simulink model "BSCForFiveAxisExperiment01"  (Simulink 8.4)
settings: Solver=ode1  StartTime=0.0  StopTime=5.122  FixedStep=0.001  RelTol=1e-3
InitFcn:
  | MainContourControlExp
values from neighbouring files (symbols this model uses):
  Acommands = DriveCommands(:,4)-HomePosDrive(4)    [MainContourControlExp.m]
  c1_i = 0.2    [MainContourControlExp.m]
  c1_j = c1_i    (= 0.2)    [MainContourControlExp.m]
  c1_k = c1_i    (= 0.2)    [MainContourControlExp.m]
  c1_x = 2    [MainContourControlExp.m]
  c1_y = c1_x    (= 2)    [MainContourControlExp.m]
  c1_z = c1_x    (= 2)    [MainContourControlExp.m]
  Ccommands = DriveCommands(:,5)-HomePosDrive(5)    [MainContourControlExp.m]
  k_i = 0.2    [MainContourControlExp.m]
  k_j = k_i    (= 0.2)    [MainContourControlExp.m]
  k_k = k_i    (= 0.2)    [MainContourControlExp.m]
  k_x = 1    [MainContourControlExp.m]
  k_y = k_x    (= 1)    [MainContourControlExp.m]
  k_z = k_x    (= 1)    [MainContourControlExp.m]
  PlantADen = [1 PlantAPara.a1 PlantAPara.a0]    [MainContourControlExp.m]
  PlantANum = [PlantAPara.b1 PlantAPara.b0]    [MainContourControlExp.m]
  PlantCDen = [1 PlantCPara.a1 PlantCPara.a0]    [MainContourControlExp.m]
  PlantCNum = [PlantCPara.b1 PlantCPara.b0]    [MainContourControlExp.m]
  PlantXDen = [1 PlantXPara.a1 PlantXPara.a0]    [MainContourControlExp.m]
  PlantXNum = [PlantXPara.b1 PlantXPara.b0]    [MainContourControlExp.m]
  PlantYDen = [1 PlantYPara.a1 PlantYPara.a0]    [MainContourControlExp.m]
  PlantYNum = [PlantYPara.b1 PlantYPara.b0]    [MainContourControlExp.m]
  PlantZDen = [1 PlantZPara.a1 PlantZPara.a0]    [MainContourControlExp.m]
  PlantZNum = [PlantZPara.b1 PlantZPara.b0]    [MainContourControlExp.m]
  R1 = 0.8    [MainContourControlExp.m]
  R2 = R1    (= 0.8)    [MainContourControlExp.m]
  R3 = R1    (= 0.8)    [MainContourControlExp.m]
  R4 = 0.8    [MainContourControlExp.m]
  R5 = R4    (= 0.8)    [MainContourControlExp.m]
  R6 = R4    (= 0.8)    [MainContourControlExp.m]
  Ts = 0.001    [MainContourControlExp.m]
  VlimitA = 5    [MainContourControlExp.m]
  VlimitC = 5    [MainContourControlExp.m]
  VlimitX = 6    [MainContourControlExp.m]
  VlimitY = 6    [MainContourControlExp.m]
  VlimitZ = 6    [MainContourControlExp.m]
  Xcommands = DriveCommands(:,1)-HomePosDrive(1)    [MainContourControlExp.m]
  Ycommands = DriveCommands(:,2)-HomePosDrive(2)    [MainContourControlExp.m]
  Zcommands = DriveCommands(:,3)-HomePosDrive(3)    [MainContourControlExp.m]
libraries: simulink x8
settings Model: Creator=Administrator  LastModifiedBy=Administrator
settings DataIOCC: SignalLoggingSaveFormat=Dataset
settings OptimizationCC: ExpressionDepthLimit=128
settings DebuggingCC: UnderspecifiedInitializationDetection=Simplified  MergeDetectMultiDrivingBlocksExec=error  FcnCallInpInsideContextMsg=EnableAllAsError  StateNameClashWarn=none
settings GRTTargetCC: CombineOutputUpdateFcns=on  GRTInterface=off

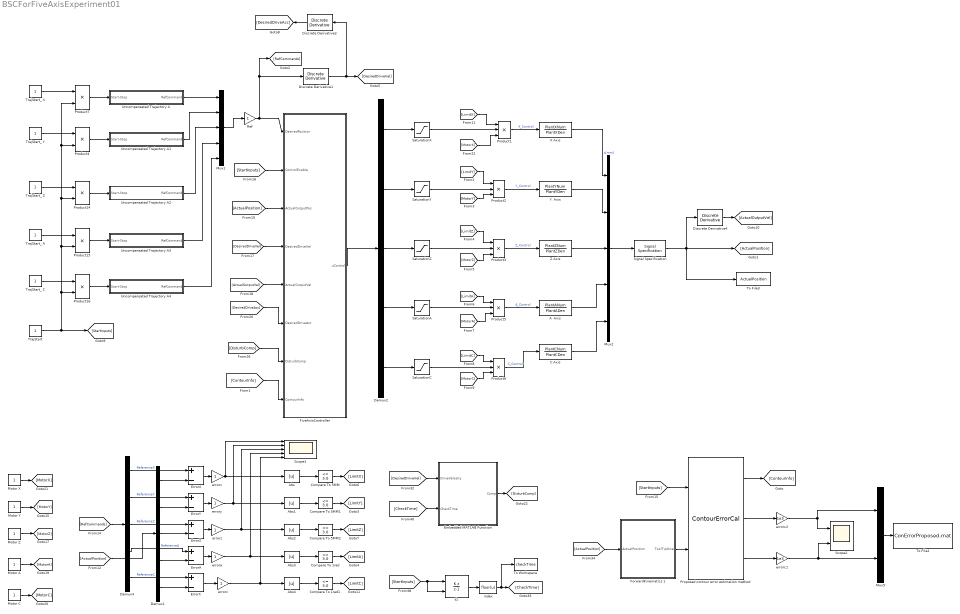
== system BSCForFiveAxisExperiment01 ==
  A  Axis : DiscreteTransferFcn  Numerator=PlantANum  Denominator=PlantADen  SampleTime=Ts
  Abs{,1..4} (5 alike) : Abs
  C Axis : DiscreteTransferFcn  Numerator=PlantCNum  Denominator=PlantCDen  SampleTime=Ts
  Compare To 1rad : simulink/Logic and Bit Operations/Compare To Constant  relop=<=  const=3.0  OutDataTypeStr=boolean
  Compare To 1rad1 : simulink/Logic and Bit Operations/Compare To Constant  relop=<=  const=3.0  OutDataTypeStr=boolean
  Compare To 5MM : simulink/Logic and Bit Operations/Compare To Constant  relop=<=  const=3.0  OutDataTypeStr=boolean
  Compare To 5MM1 : simulink/Logic and Bit Operations/Compare To Constant  relop=<=  const=3.0  OutDataTypeStr=boolean
  Compare To 5MM2 : simulink/Logic and Bit Operations/Compare To Constant  relop=<=  const=3.0  OutDataTypeStr=boolean
  Demux1 : Demux  Outputs=5
  Demux2 : Demux  Outputs=5
  Demux4 : Demux  Outputs=5
  Discrete Derivative1 : simulink/Discrete/Discrete Derivative  gainval=1.0  ICPrevScaledInput=0.0  InputProcessing=Inherited  OutMin=[]  OutMax=[]  OutDataType=fixdt(1, 16)  OutScaling=2^-10  DoSatur=off
  Discrete Derivative2 : simulink/Discrete/Discrete Derivative  gainval=1.0  ICPrevScaledInput=0.0  InputProcessing=Inherited  OutMin=[]  OutMax=[]  OutDataType=fixdt(1, 16)  OutScaling=2^-10  DoSatur=off
  Discrete Derivative4 : simulink/Discrete/Discrete Derivative  gainval=1.0  ICPrevScaledInput=0.0  InputProcessing=Inherited  OutMin=[]  OutMax=[]  OutDataType=fixdt(1, 16)  OutScaling=2^-10  DoSatur=off
  Embedded MATLAB Function : MATLAB Function  TreatAsAtomicUnit=on
  ErrorA : Sum  Inputs=+-
  ErrorC : Sum  Inputs=+-
  ErrorX : Sum  Inputs=+-
  ErrorY : Sum  Inputs=+-
  ErrorZ : Sum  Inputs=+-
  FiveAxisController : MATLAB Function  TreatAsAtomicUnit=on
  ForwardKinematics 1 : MATLAB Function  TreatAsAtomicUnit=on
  Motor A : Constant
  Motor C : Constant
  Motor X : Constant
  Motor Y : Constant
  Motor Z : Constant
  Mux1 : Mux  Inputs=5
  Mux2 : Mux  Inputs=5
  Mux5 : Mux  Inputs=2
  Product{1..3,5..6} (5 alike) : Product  Inputs=3  RndMeth=Zero
  Product{4,7,14..16} (5 alike) : Product  SampleTime=Ts  RndMeth=Zero
  Proposed contour error estimation method : S-Function  FunctionName=ContourErrorCal  Parameters=X Y Z I J K U  EnableBusSupport=off
  "Ref " : Gain  SampleTime=0.001
  SaturationA : Saturate  UpperLimit=VlimitA  LowerLimit=-VlimitA
  SaturationC : Saturate  UpperLimit=VlimitC  LowerLimit=-VlimitC
  SaturationX : Saturate  UpperLimit=VlimitX  LowerLimit=-VlimitX
  SaturationY : Saturate  UpperLimit=VlimitY  LowerLimit=-VlimitY
  SaturationZ : Saturate  UpperLimit=VlimitZ  LowerLimit=-VlimitZ
  Scope1 : Scope  NumInputPorts=5
      settings: TimeRange=5.122  YMin=-0.1~-0.04~-0.04~-0.001~-0.0015  YMax=0.1~0.06~0.06~0.001~0.0015  SaveName=ScopeData2  MaxDataPoints=5122
  Scope2 : Scope  NumInputPorts=2
      settings: YMin=0~0  YMax=90~1.2  SaveName=ScopeData3
  Signal Specification : SignalSpecification  Dimensions=5
  To File2 : ToFile  Filename=ConErrorProposed.mat  MatrixName=Proposed
  To File3 : ToFile  Filename=ActualPosition  MatrixName=ActualPos
  To Workspace : ToWorkspace  VariableName=checkTime  SampleTime=-1
  TrajStart : Constant
  TrajStart_ A : Constant
  TrajStart_ C : Constant
  "TrajStart_ X " : Constant
  TrajStart_ Y : Constant
  TrajStart_ Z : Constant
  Uncompensated Trajectory A : Subsystem
  Uncompensated Trajectory A1 : Subsystem
  Uncompensated Trajectory A2 : Subsystem
  Uncompensated Trajectory A3 : Subsystem
  Uncompensated Trajectory A4 : Subsystem
  "X Axis " : DiscreteTransferFcn  Numerator=PlantXNum  Denominator=PlantXDen  SampleTime=Ts
  Y  Axis : DiscreteTransferFcn  Numerator=PlantYNum  Denominator=PlantYDen  SampleTime=Ts
  Z Axis : DiscreteTransferFcn  Numerator=PlantZNum  Denominator=PlantZDen  SampleTime=Ts
  errora : Gain  SampleTime=0.001
  errorc : Gain  SampleTime=0.001
  errorc1 : Gain  Gain=1e3  SampleTime=0.001
  errorc2 : Gain  Gain=1e3  SampleTime=0.001
  errorx : Gain  SampleTime=0.001
  errory : Gain  SampleTime=0.001
  errorz : Gain  SampleTime=0.001
  index : Fcn  Expr=floor(u)
  t1 : DiscreteIntegrator  IntegratorMethod=Accumulation: Backward Euler  ExternalReset=rising  SampleTime=Ts
  wires:
  TrajStart/1 -> [StartInputs], Product16/2, Product15/2, Product14/2, Product7/2, Product4/2
  SaturationX/1 -> Product1/2
  [LimitX] -> Product1/1
  [MotorX] -> Product1/3
  Product1/1 -> "X Axis "/1  "X_Control"
  Mux1/1 -> "Ref "/1
  SaturationY/1 -> Product2/2
  [LimitY] -> Product2/1
  [MotorY] -> Product2/3
  Product2/1 -> Y  Axis/1  "Y_Control"
  SaturationZ/1 -> Product3/2
  [LimitZ] -> Product3/1
  [MotorZ] -> Product3/3
  Product3/1 -> Z Axis/1  "Z_Control"
  SaturationA/1 -> Product5/2
  [LimitA] -> Product5/1
  [MotorA] -> Product5/3
  Product5/1 -> A  Axis/1  "A_Control"
  SaturationC/1 -> Product6/2
  [LimitC] -> Product6/1
  [MotorC] -> Product6/3
  Product6/1 -> C Axis/1  "C_Control"
  Compare To 5MM/1 -> [LimitX]
  Abs/1 -> Compare To 5MM/1
  Compare To 5MM1/1 -> [LimitY]
  Abs1/1 -> Compare To 5MM1/1
  ErrorY/1 -> errory/1
  Demux1/1 -> ErrorX/2
  Demux1/2 -> ErrorY/2
  Demux4/1 -> ErrorX/1  "ReferenceX"
  Demux4/2 -> ErrorY/1  "ReferenceY"
  [RefCommands] -> Demux4/1
  Compare To 5MM2/1 -> [LimitZ]
  Abs2/1 -> Compare To 5MM2/1
  ErrorZ/1 -> errorz/1
  Demux1/3 -> ErrorZ/2
  Demux4/3 -> ErrorZ/1  "ReferenceZ"
  Compare To 1rad/1 -> [LimitA]
  Abs3/1 -> Compare To 1rad/1
  Demux1/4 -> ErrorA/2
  Demux4/4 -> ErrorA/1  "ReferenceA"
  Compare To 1rad1/1 -> [LimitC]
  Abs4/1 -> Compare To 1rad1/1
  ErrorC/1 -> errorc/1
  Demux1/5 -> ErrorC/2
  Demux4/5 -> ErrorC/1  "ReferenceC"
  [ActualPosition] -> Demux1/1
  Discrete Derivative1/1 -> [DesiredDriveVel], Discrete Derivative2/1
  Discrete Derivative2/1 -> [DesiredDriveAcc]
  t1/1 -> index/1
  [StartInputs] -> t1/1, t1/2
  index/1 -> To Workspace/1, [CheckTime]
  Embedded MATLAB Function/1(Comp) -> [DisturbComp]
  [DesiredDriveVel] -> Embedded MATLAB Function/1(DriveVelosity)
  [CheckTime] -> Embedded MATLAB Function/2(CheckTime)
  ErrorA/1 -> errora/1
  ErrorX/1 -> errorx/1
  "TrajStart_ X "/1 -> Product7/1
  "Ref "/1 -> [RefCommands], Discrete Derivative1/1, FiveAxisController/1(DesiredPosition)
  errorx/1 -> Scope1/1, Abs/1
  errory/1 -> Scope1/2, Abs1/1
  errorz/1 -> Scope1/3, Abs2/1
  errora/1 -> Scope1/4, Abs3/1
  errorc/1 -> Scope1/5, Abs4/1
  Product7/1 -> Uncompensated Trajectory A/1(Start-Stop)
  Product4/1 -> Uncompensated Trajectory A1/1(Start-Stop)
  Product14/1 -> Uncompensated Trajectory A2/1(Start-Stop)
  Product15/1 -> Uncompensated Trajectory A3/1(Start-Stop)
  TrajStart_ Y/1 -> Product4/1
  TrajStart_ Z/1 -> Product14/1
  TrajStart_ A/1 -> Product15/1
  TrajStart_ C/1 -> Product16/1
  Product16/1 -> Uncompensated Trajectory A4/1(Start-Stop)
  Uncompensated Trajectory A3/1(RefCommand) -> Mux1/4
  Uncompensated Trajectory A/1(RefCommand) -> Mux1/1
  Uncompensated Trajectory A1/1(RefCommand) -> Mux1/2
  Uncompensated Trajectory A2/1(RefCommand) -> Mux1/3
  Uncompensated Trajectory A4/1(RefCommand) -> Mux1/5
  [StartInputs] -> FiveAxisController/2(ControlEnable)
  [ActualPosition] -> FiveAxisController/3(ActualOutputPos)
  [DesiredDriveVel] -> FiveAxisController/4(DesiredDriveVel)
  [DesiredDriveAcc] -> FiveAxisController/6(DesiredDriveAcc)
  [ActualOutputVel] -> FiveAxisController/5(ActualOutputVel)
  [DisturbComp] -> FiveAxisController/7(DisturbComp)
  [ContourInfo] -> FiveAxisController/8(ContourInfo)
  FiveAxisController/1(uControl) -> Demux2/1
  Demux2/5 -> SaturationC/1
  Demux2/4 -> SaturationA/1
  Demux2/3 -> SaturationZ/1
  Demux2/2 -> SaturationY/1
  Demux2/1 -> SaturationX/1
  Discrete Derivative4/1 -> [ActualOutputVel]
  Mux2/1 -> Signal Specification/1
  Signal Specification/1 -> Discrete Derivative4/1, To File3/1, [ActualPosition]
  "X Axis "/1 -> Mux2/1  "x[mm]"
  Y  Axis/1 -> Mux2/2
  Z Axis/1 -> Mux2/3
  A  Axis/1 -> Mux2/4
  C Axis/1 -> Mux2/5
  Motor Y/1 -> [MotorY]
  Motor X/1 -> [MotorX]
  Motor Z/1 -> [MotorZ]
  Motor A/1 -> [MotorA]
  Motor C/1 -> [MotorC]
  [StartInputs] -> Proposed contour error estimation method/1
  ForwardKinematics 1/1(ToolTipOrien) -> Proposed contour error estimation method/2
  Proposed contour error estimation method/1 -> [ContourInfo]
  [ActualPosition] -> ForwardKinematics 1/1(ActualPosition)
  Proposed contour error estimation method/2 -> errorc2/1
  Proposed contour error estimation method/3 -> errorc1/1
  Mux5/1 -> To File2/1
  errorc2/1 -> Mux5/1, Scope2/1
  errorc1/1 -> Mux5/2, Scope2/2

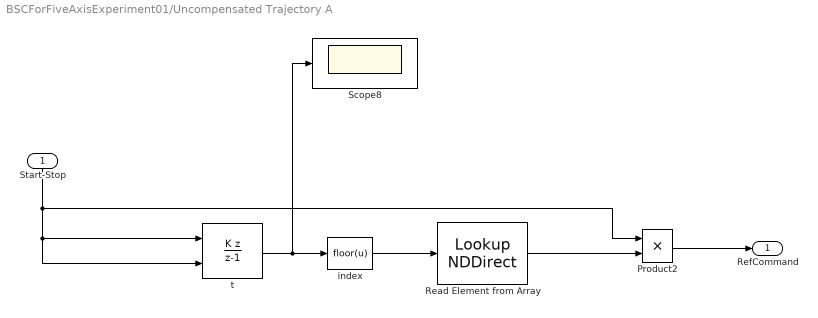
== system BSCForFiveAxisExperiment01/Uncompensated Trajectory A ==
  Start-Stop : Inport
  Product2 : Product  RndMeth=Zero
  Read Element from Array : LookupNDDirect  NumberOfTableDimensions=1  Table=Xcommands
  Scope8 : Scope
  index : Fcn  Expr=floor(u)
  t : DiscreteIntegrator  IntegratorMethod=Accumulation: Backward Euler  ExternalReset=rising  SampleTime=Ts
  RefCommand : Outport
  wires:
  Read Element from Array/1 -> Product2/2
  t/1 -> Scope8/1, index/1
  Product2/1 -> RefCommand/1
  Start-Stop/1 -> Product2/1, t/1, t/2
  index/1 -> Read Element from Array/1

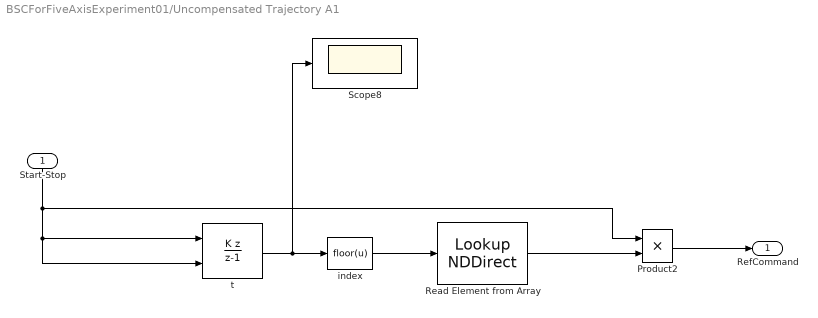
== system BSCForFiveAxisExperiment01/Uncompensated Trajectory A1 ==
  Start-Stop : Inport
  Product2 : Product  RndMeth=Zero
  Read Element from Array : LookupNDDirect  NumberOfTableDimensions=1  Table=Ycommands
  Scope8 : Scope
  index : Fcn  Expr=floor(u)
  t : DiscreteIntegrator  IntegratorMethod=Accumulation: Backward Euler  ExternalReset=rising  SampleTime=Ts
  RefCommand : Outport
  wires:
  index/1 -> Read Element from Array/1
  Start-Stop/1 -> t/2, t/1, Product2/1
  Product2/1 -> RefCommand/1
  t/1 -> index/1, Scope8/1
  Read Element from Array/1 -> Product2/2

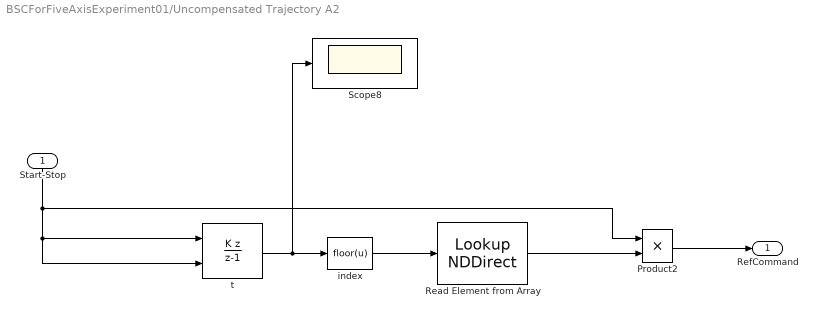
== system BSCForFiveAxisExperiment01/Uncompensated Trajectory A2 ==
  Start-Stop : Inport
  Product2 : Product  RndMeth=Zero
  Read Element from Array : LookupNDDirect  NumberOfTableDimensions=1  Table=Zcommands
  Scope8 : Scope
  index : Fcn  Expr=floor(u)
  t : DiscreteIntegrator  IntegratorMethod=Accumulation: Backward Euler  ExternalReset=rising  SampleTime=Ts
  RefCommand : Outport
  wires:
  Read Element from Array/1 -> Product2/2
  t/1 -> Scope8/1, index/1
  Product2/1 -> RefCommand/1
  Start-Stop/1 -> Product2/1, t/1, t/2
  index/1 -> Read Element from Array/1

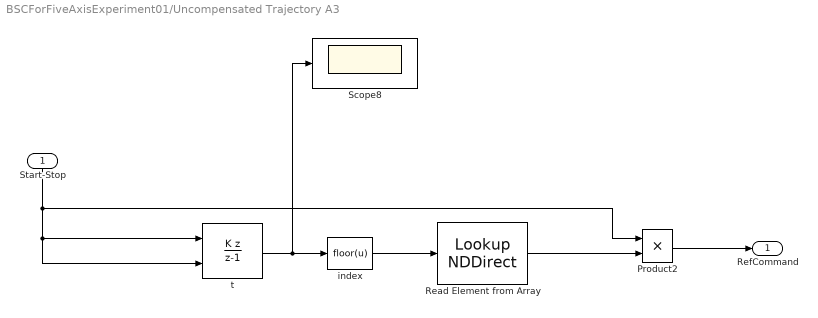
== system BSCForFiveAxisExperiment01/Uncompensated Trajectory A3 ==
  Start-Stop : Inport
  Product2 : Product  RndMeth=Zero
  Read Element from Array : LookupNDDirect  NumberOfTableDimensions=1  Table=Acommands
  Scope8 : Scope
  index : Fcn  Expr=floor(u)
  t : DiscreteIntegrator  IntegratorMethod=Accumulation: Backward Euler  ExternalReset=rising  SampleTime=Ts
  RefCommand : Outport
  wires:
  index/1 -> Read Element from Array/1
  Start-Stop/1 -> t/2, t/1, Product2/1
  Product2/1 -> RefCommand/1
  t/1 -> index/1, Scope8/1
  Read Element from Array/1 -> Product2/2

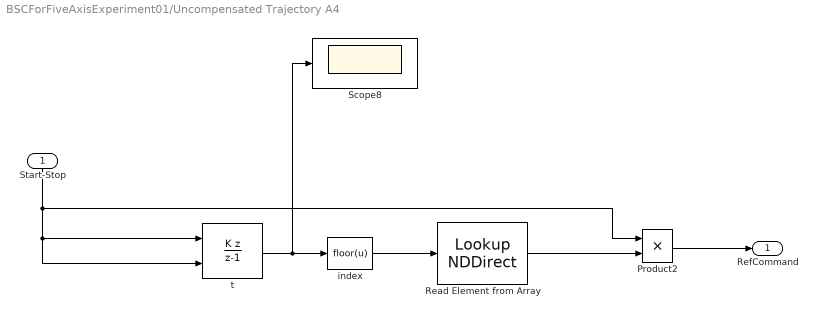
== system BSCForFiveAxisExperiment01/Uncompensated Trajectory A4 ==
  Start-Stop : Inport
  Product2 : Product  RndMeth=Zero
  Read Element from Array : LookupNDDirect  NumberOfTableDimensions=1  Table=Ccommands
  Scope8 : Scope
  index : Fcn  Expr=floor(u)
  t : DiscreteIntegrator  IntegratorMethod=Accumulation: Backward Euler  ExternalReset=rising  SampleTime=Ts
  RefCommand : Outport
  wires:
  Read Element from Array/1 -> Product2/2
  t/1 -> Scope8/1, index/1
  Product2/1 -> RefCommand/1
  Start-Stop/1 -> Product2/1, t/1, t/2
  index/1 -> Read Element from Array/1

== matlab function FiveAxisController ==
  data: DesiredPosition input double; ControlEnable input double; ActualOutputPos input double; DesiredDriveVel input double; ActualOutputVel input double size=[5 1]; DesiredDriveAcc input double; uControl output double; DisturbComp input double; ContourInfo input double; c1_x parameter double; k_x parameter double; c1_y parameter double; k_y parameter double; c1_z parameter double; k_z parameter double; c1_i parameter double; k_i parameter double; c1_j parameter double; k_j parameter double; c1_k parameter double; k_k parameter double; R1 parameter double; R2 parameter double; R3 parameter double; R4 parameter double; R5 parameter double; R6 parameter double
function uControl = BSC(DesiredPosition,ControlEnable,ActualOutputPos,DesiredDriveVel,ActualOutputVel,DesiredDriveAcc,DisturbComp,ContourInfo,c1_x,k_x,c1_y,k_y,c1_z,k_z,c1_i,k_i,c1_j,k_j,c1_k,k_k,R1,R2,R3,R4,R5,R6)

%% persistent variables
persistent PlantX PlantY PlantZ PlantA PlantC
% Plant parameters,three-axis experimental platform
if isempty(PlantX)
    PlantXCom=struct('J',0.00009537,'B',0.0007158,'Ka',0.8268,'Kt',0.512,'rg',10/(2*pi));   
    %PlantXCom=struct('J',0.00004333,'B',0.00009417,'Ka',0.8268,'Kt',0.512,'rg',10/(2*pi));    
    PlantX=struct('K',0,'m',0,'c',0);
    PlantX.K = PlantXCom.Ka*PlantXCom.Kt*PlantXCom.rg;   %(N*m^2/V)/1000
    PlantX.m = PlantXCom.J/PlantX.K; %(V*s^2/mm) 
    PlantX.c = PlantXCom.B/PlantX.K; %(V*s/mm)
end
if isempty(PlantY)
    PlantYCom=struct('J',0.0001332,'B',0.0004852,'Ka',0.8268,'Kt',0.512,'rg',10/(2*pi));  
    %PlantYCom=struct('J',0.00004333,'B',0.00009417,'Ka',0.8268,'Kt',0.512,'rg',10/(2*pi));  
    PlantY=struct('K',0,'m',0,'c',0);    
    PlantY.K = PlantYCom.Ka*PlantYCom.Kt*PlantYCom.rg; %(N*m^2/V)/1000
    PlantY.m = PlantYCom.J/PlantY.K; %(V*s^2/mm)
    PlantY.c = PlantYCom.B/PlantY.K; %(V*s/mm)
end
if isempty(PlantZ)
    PlantZCom=struct('J',0.0001006,'B',0.0002758,'Ka',0.8268,'Kt',0.512,'rg',10/(2*pi));  
    %PlantZCom=struct('J',0.00004367,'B',0.00009155,'Ka',0.8268,'Kt',0.512,'rg',10/(2*pi));
    PlantZ=struct('K',0,'m',0,'c',0);
    PlantZ.K = PlantZCom.Ka*PlantZCom.Kt*PlantZCom.rg; %(N*m^2/V)/1000
    PlantZ.m = PlantZCom.J/PlantZ.K; %(V*s^2/mm)
    PlantZ.c = PlantZCom.B/PlantZ.K; %(V*s/mm)
end
if isempty(PlantA)
    PlantACom=struct('J',0.00004333,'B',0.00009417,'Ka',0.8268,'Kt',0.512,'rg',1/100);
    PlantA=struct('K',0,'m',0,'c',0);
    PlantA.K = PlantACom.Ka*PlantACom.Kt*PlantACom.rg;
    PlantA.m = PlantACom.J/PlantA.K; %(V*s^2/rad)
    PlantA.c = PlantACom.B/PlantA.K; %(V*s/rad)
end
if isempty(PlantC)
    PlantCCom=struct('J',0.00004367,'B',0.00009155,'Ka',0.8268,'Kt',0.512,'rg',1/100);
    PlantC=struct('K',0,'m',0,'c',0);
    PlantC.K = PlantCCom.Ka*PlantCCom.Kt*PlantCCom.rg;
    PlantC.m = PlantCCom.J/PlantC.K; %(V*s^2/rad)
    PlantC.c = PlantCCom.B/PlantC.K; %(V*s/rad)
end

M = diag([PlantX.m PlantY.m PlantZ.m PlantA.m PlantC.m]);   
C = diag([PlantX.c PlantY.c PlantZ.c PlantA.c PlantC.c]);

%% This parameter is used for simuliation for the fan tool path

%% -----------------------------------------------------------------------------------------------------------------------
% This code is used for sliding mode control for five-axis machine tool 
if ControlEnable == 1  
    % Design the tracking controller by using backstepping controlller 
    % 获取并计算轨迹规划点和实际运动点
    desiredAxisPos = DesiredPosition(1:5);                                 % desiredAxisPos = [x y z a c]      关节空间期望位置量
    acutalAxisPos  = ActualOutputPos(1:5);                                 % ( 5 X 1 )   关节空间实际位置量
    desiredTaskPos = ForwardKinematics(desiredAxisPos);                    % desiredTaskPos = [x y z i j k]    操作空间期望位置量
    actualTaskPos  = ForwardKinematics(acutalAxisPos);                     % ( 6 X 1 )   操作空间实际位置量
    
    desiredJocMatrix = Jacobin(desiredAxisPos);                            % ( 6 X 5 )   期望位置的雅克比矩阵
    actualJocMatrix  = Jacobin(acutalAxisPos);                             % ( 6 X 5 )   实际位置的雅克比矩阵
    desiredAxisVel   = DesiredDriveVel(1:5);                               % ( 5 X 1 )   关节空间期望速度量
    actualAxisVel    = ActualOutputVel(1:5);                               % ( 5 X 1 )   关节空间实际速度量 
    desiredTaskVel   = desiredJocMatrix * desiredAxisVel;                  %             操作空间期望速度量          
    actualTaskVel    = actualJocMatrix * actualAxisVel;                    %             操作空间实际速度量

    desiredJocMatrixDer1 = JacobinDer1(desiredAxisPos,desiredAxisVel);                                 % 期望位置的海瑟矩阵 雅克比一阶导
    desiredAxisAcc       = DesiredDriveAcc(1:5);                                                       % 关节空间的期望加速度量
    desiredTaskAcc       = desiredJocMatrixDer1*desiredAxisVel + desiredJocMatrix*desiredAxisAcc;      % 操作空间的期望加速度量
    actualJocMatrixDer1  = JacobinDer1(acutalAxisPos,actualAxisVel);                                   % 实际位置的海瑟矩阵 雅克比一阶导

    % 利用规划点和实际点位置求取位置跟踪误差和速度跟踪误差
    TrackingPositionErrorX = desiredTaskPos(1) - actualTaskPos(1);
    TrackingPositionErrorY = desiredTaskPos(2) - actualTaskPos(2);
    TrackingPositionErrorZ = desiredTaskPos(3) - actualTaskPos(3);
    TrackingPositionErrorI = desiredTaskPos(4) - actualTaskPos(4);
    TrackingPositionErrorJ = desiredTaskPos(5) - actualTaskPos(5);
    TrackingPositionErrorK = desiredTaskPos(6) - actualTaskPos(6);
    
    TrackingVelocityErrorX =  desiredTaskVel(1) - actualTaskVel(1);      
    TrackingVelocityErrorY =  desiredTaskVel(2) - actualTaskVel(2);   
    TrackingVelocityErrorZ =  desiredTaskVel(3) - actualTaskVel(3);   
    TrackingVelocityErrorI =  desiredTaskVel(4) - actualTaskVel(4);   
    TrackingVelocityErrorJ =  desiredTaskVel(5) - actualTaskVel(5);   
    TrackingVelocityErrorK =  desiredTaskVel(6) - actualTaskVel(6);   
    
    % 获取轮廓误差估计分量零一二阶导数 ContourInfo（1-18）
    ContourErrorXDer2 = ContourInfo(13);
    ContourErrorYDer2 = ContourInfo(14);
    ContourErrorZDer2 = ContourInfo(15);
    ContourErrorIDer2 = ContourInfo(16);
    ContourErrorJDer2 = ContourInfo(17);
    ContourErrorKDer2 = ContourInfo(18);
    ContourErrorDer2 = [ContourErrorXDer2 ContourErrorYDer2 ContourErrorZDer2 ContourErrorIDer2 ContourErrorJDer2 ContourErrorKDer2]';
    
    % 设定未知参数 Aerfal 和 Z2
    Z1_x = TrackingPositionErrorX + R1*ContourInfo(1);
    Z1_y = TrackingPositionErrorY + R1*ContourInfo(2);
    Z1_z = TrackingPositionErrorZ + R1*ContourInfo(3);
    Z1_i = TrackingPositionErrorI + R1*ContourInfo(4);
    Z1_j = TrackingPositionErrorJ + R1*ContourInfo(5);
    Z1_k = TrackingPositionErrorK + R1*ContourInfo(6);
    Z1 = [Z1_x Z1_y Z1_z Z1_i Z1_j Z1_k]';    

    Z1Der1_x = TrackingVelocityErrorX + R1*ContourInfo(7);
    Z1Der1_y = TrackingVelocityErrorY + R1*ContourInfo(8);
    Z1Der1_z = TrackingVelocityErrorZ + R1*ContourInfo(9);
    Z1Der1_i = TrackingVelocityErrorI + R1*ContourInfo(10);
    Z1Der1_j = TrackingVelocityErrorJ + R1*ContourInfo(11);
    Z1Der1_k = TrackingVelocityErrorK + R1*ContourInfo(12);
    Z1Der1 = [Z1Der1_x Z1Der1_y Z1Der1_z Z1Der1_i Z1Der1_j Z1Der1_k]';

    R = diag([R1 R2 R3 R4 R5 R6]);
    C1 = diag([c1_x c1_y c1_z c1_i c1_j c1_k]);
    K = diag([k_x k_y k_z k_i k_j k_k]);
    
    % Calculate the control input for each drive
    uControl = M*pinv(actualJocMatrix)*(desiredTaskAcc + R*ContourErrorDer2 + C1*Z1Der1 + K*Z1Der1 + K*C1*Z1 - actualJocMatrixDer1*actualAxisVel) + C*actualAxisVel + DisturbComp;

else
    uControl = [0 0 0 0 0]';
end
end


%%
function TipOrien = ForwardKinematics(DriveCommands)

Lacy = 0;
Lacz = 41;

HomePosDrive=[113.232633012931,18.4363460319427,0.239716132104988,0.686766850928449,-0.169983380596482];
% HomePosDrive=[0,0,0,0,0];

X = DriveCommands(1)+HomePosDrive(1);
Y = DriveCommands(2)+HomePosDrive(2);
Z = DriveCommands(3)+HomePosDrive(3);
A = DriveCommands(4)+HomePosDrive(4);
C = DriveCommands(5)+HomePosDrive(5);


Oi = sin(A)*sin(C);
Oj = sin(A)*cos(C);
Ok = cos(A);
Px = cos(C)*X+cos(A)*sin(C)*Y+sin(A)*sin(C)*Z-cos(A)*sin(C)*Lacy-sin(A)*sin(C)*Lacz;
Py = -sin(C)*X+cos(A)*cos(C)*Y+sin(A)*cos(C)*Z+(1-cos(A)*cos(C))*Lacy-sin(A)*cos(C)*Lacz;
Pz = -sin(A)*Y+cos(A)*Z+sin(A)*Lacy+(1-cos(A))*Lacz;

TipOrien = [Px Py Pz Oi Oj Ok]';
end

function J = Jacobin(DriveCommands)

Lacy = 0;
Lacz = 41;

HomePosDrive=[113.232633012931,18.4363460319427,0.239716132104988,0.686766850928449,-0.169983380596482];
%HomePosDrive=[0,0,0,0,0];

X = DriveCommands(1)+HomePosDrive(1);
Y = DriveCommands(2)+HomePosDrive(2);
Z = DriveCommands(3)+HomePosDrive(3);
A = DriveCommands(4)+HomePosDrive(4);
C = DriveCommands(5)+HomePosDrive(5);

 
J = [   cos(C)  cos(A)*sin(C)    sin(A)*sin(C)        -sin(A)*sin(C)*Y+cos(A)*sin(C)*Z+sin(A)*sin(C)*Lacy-cos(A)*sin(C)*Lacz     -sin(C)*X+cos(A)*cos(C)*Y+sin(A)*cos(C)*Z-cos(A)*cos(C)*Lacy-sin(A)*cos(C)*Lacz
       -sin(C)   cos(A)*cos(C)    sin(A)*cos(C)       -sin(A)*cos(C)*Y+cos(A)*cos(C)*Z+sin(A)*cos(C)*Lacy-cos(A)*cos(C)*Lacz     -cos(C)*X-cos(A)*sin(C)*Y-sin(A)*sin(C)*Z+cos(A)*sin(C)*Lacy+sin(A)*sin(C)*Lacz
       0          -sin(A)            cos(A)                 -cos(A)*Y-sin(A)*Z+cos(A)*Lacy+sin(A)*Lacz                                           0
       0            0                  0                                  cos(A)*sin(C)                                                     sin(A)*cos(C)
       0            0                  0                                  cos(A)*cos(C)                                                     -sin(A)*sin(C)
       0            0                  0                                     -sin(A)                                                             0  ];


end

function JDer1 = JacobinDer1(PositionCommands,VelosityCommands)

Lacy = 0;
Lacz = 41;

HomePosDrive=[113.232633012931,18.4363460319427,0.239716132104988,0.686766850928449,-0.169983380596482];
%HomePosDrive=[0,0,0,0,0];

X = PositionCommands(1)+HomePosDrive(1);
Y = PositionCommands(2)+HomePosDrive(2);
Z = PositionCommands(3)+HomePosDrive(3);
A = PositionCommands(4)+HomePosDrive(4);
C = PositionCommands(5)+HomePosDrive(5);

XDer1 = VelosityCommands(1);
YDer1 = VelosityCommands(2);
ZDer1 = VelosityCommands(3);
ADer1 = VelosityCommands(4);
CDer1 = VelosityCommands(5);

JDer111 = -sin(C)*CDer1;
JDer112 = -sin(A)*sin(C)*ADer1+cos(A)*cos(C)*CDer1;
JDer113 = cos(A)*sin(C)*ADer1+sin(A)*cos(C)*CDer1;
JDer114=-sin(A)*sin(C)*YDer1+cos(A)*sin(C)*ZDer1-cos(A)*sin(C)*Y*ADer1-sin(A)*sin(C)*Z*ADer1+cos(A)*sin(C)*Lacy*ADer1+sin(A)*sin(C)*Lacz*ADer1-...
   sin(A)*cos(C)*Y*CDer1+cos(A)*cos(C)*Z*CDer1+sin(A)*cos(C)*Lacy*CDer1-cos(A)*cos(C)*Lacz*CDer1;
JDer115=-sin(C)*XDer1+cos(A)*cos(C)*YDer1+sin(A)*cos(C)*ZDer1-sin(A)*cos(C)*Y*ADer1+cos(A)*cos(C)*Z*ADer1+sin(A)*cos(C)*Lacy*ADer1-cos(A)*cos(C)*Lacz*ADer1-...
   cos(C)*X*CDer1-cos(A)*sin(C)*Y*CDer1-sin(A)*sin(C)*Z*CDer1+cos(A)*sin(C)*Lacy*CDer1+sin(A)*sin(C)*Lacz*CDer1;

JDer121 = -cos(C)*CDer1;
JDer122 = -sin(A)*cos(C)*ADer1-cos(A)*sin(C)*CDer1;
JDer123 = cos(A)*cos(C)*ADer1-sin(A)*sin(C)*CDer1;
JDer124=-sin(A)*cos(C)*YDer1+cos(A)*cos(C)*ZDer1-cos(A)*cos(C)*Y*ADer1-sin(A)*cos(C)*Z*ADer1+cos(A)*cos(C)*Lacy*ADer1+sin(A)*cos(C)*Lacz*ADer1+...
   sin(A)*sin(C)*Y*CDer1-cos(A)*sin(C)*Z*CDer1-sin(A)*sin(C)*Lacy*CDer1+cos(A)*sin(C)*Lacz*CDer1;
JDer125=-cos(C)*XDer1-cos(A)*sin(C)*YDer1-sin(A)*sin(C)*ZDer1+sin(A)*sin(C)*Y*ADer1-cos(A)*sin(C)*Z*ADer1-sin(A)*sin(C)*Lacy*ADer1+cos(A)*sin(C)*Lacz*ADer1+...
    sin(C)*X*CDer1-cos(A)*cos(C)*Y*CDer1-sin(A)*cos(C)*Z*CDer1+cos(A)*cos(C)*Lacy*CDer1+sin(A)*cos(C)*Lacz*CDer1;

JDer131 = 0;
JDer132 = -cos(A)*ADer1;
JDer133 = -sin(A)*ADer1;
JDer134=-cos(A)*YDer1-sin(A)*ZDer1+sin(A)*Y*ADer1-cos(A)*Z*ADer1-sin(A)*Lacy*ADer1+cos(A)*Lacz*ADer1;
JDer135=0;

JDer144 = -sin(A)*sin(C)*ADer1+cos(A)*cos(C)*CDer1;
JDer145 = cos(A)*cos(C)*ADer1-sin(A)*sin(C)*CDer1;

JDer154 = -sin(A)*cos(C)*ADer1-cos(A)*sin(C)*CDer1;
JDer155 = -cos(A)*sin(C)*ADer1-sin(A)*cos(C)*CDer1;

JDer164 = -cos(A)*ADer1;
JDer165 = 0;


JDer1 = [ JDer111  JDer112    JDer113    JDer114     JDer115
          JDer121  JDer122    JDer123    JDer124     JDer125
          JDer131  JDer132    JDer133    JDer134     JDer135
            0          0            0    JDer144     JDer145    
            0          0            0    JDer154     JDer155
            0          0            0    JDer164     JDer165];
end

== matlab function Embedded MATLAB Function ==
  data: DriveVelosity input double; Comp output double; CheckTime input double
function Comp=Disturb(DriveVelosity,CheckTime)

% Set the condition for choosing simulink mode or real time control mode
if (CheckTime>=0 && CheckTime<=5122)
    if (DriveVelosity(1)>0)
%         XComp=0.87880;
        XComp=0;
    elseif (DriveVelosity(1)<0)
%         XComp=-0.94645;
        XComp=0;        
    else
        XComp=0;
    end

    if (DriveVelosity(2)>0)
%         YComp=1.10784;
        YComp=0;
    elseif (DriveVelosity(2)<0)
%         YComp=-1.04272;
        YComp=0;
    else
        YComp=0;
    end

    if (DriveVelosity(3)>0)
%         ZComp=0.84693;
        ZComp=0;       
    elseif (DriveVelosity(3)<0)
%         ZComp=-0.40211;
        ZComp=0;        
    else
        ZComp=0;
    end

    if (DriveVelosity(4)>0)
%         AComp=0.43188;
        AComp=0;
    elseif (DriveVelosity(4)<0)
%         AComp=-0.40411;
        AComp=0;
    else
        AComp=0;
    end

    if (DriveVelosity(5)>0)
%         CComp=0.99398;
        CComp=0;
    elseif (DriveVelosity(5)<0)
%         CComp=-0.97750;
        CComp=0;
    else
        CComp=0;
    end
    Comp=[XComp YComp ZComp AComp CComp]';
else
    XComp=0;
    YComp=0;
    ZComp=0;
    AComp=0;
    CComp=0;
    Comp=[XComp YComp ZComp AComp CComp]';    
end
end

== matlab function ForwardKinematics 1 ==
  data: ActualPosition input double; ToolTipOrien output double; HomePosDrive parameter double
function ToolTipOrien=ForwardKinematics(ActualPosition,HomePosDrive)

Lacy = 0;
Lacz = 41;

X = ActualPosition(1)+HomePosDrive(1);
Y = ActualPosition(2)+HomePosDrive(2);
Z = ActualPosition(3)+HomePosDrive(3);
A = ActualPosition(4)+HomePosDrive(4);
C = ActualPosition(5)+HomePosDrive(5);

Px = cos(C)*X+cos(A)*sin(C)*Y+sin(A)*sin(C)*Z-cos(A)*sin(C)*Lacy-sin(A)*sin(C)*Lacz;
Py = -sin(C)*X+cos(A)*cos(C)*Y+sin(A)*cos(C)*Z+(1-cos(A)*cos(C))*Lacy-sin(A)*cos(C)*Lacz;
Pz = -sin(A)*Y+cos(A)*Z+sin(A)*Lacy+(1-cos(A))*Lacz;

Oi = sin(A)*sin(C);
Oj = sin(A)*cos(C);
Ok = cos(A);

ToolTipOrien=[Px Py Pz Oi Oj Ok A C]';
end
